simulink model "teach_from_joints"  (R2021a)
settings: Solver=FixedStepAuto  StartTime=0.0  StopTime=1000  FixedStep=SAMPLE_TIME  RelTol=1e-3
values from neighbouring files (symbols this model uses):
  dh_a = dh_list(:,3)    [move_joints_setup.m]
  dh_alpha = dh_list(:,4)    [move_joints_setup.m]
  dh_d = dh_list(:,2)+[0 0 0 0 0 length_f2t]'    [move_joints_setup.m]
  dh_theta_offset = dh_list(:,1)    [move_joints_setup.m]
  init_position = [274.5 0 543.1-138]    [move_joints_setup.m]
  initial_q = [0, 0, 0, 0, pi/2, 0]    [move_joints_setup.m]
  SAMPLE_TIME = 0.004    [move_joints_setup.m]
  theta_acc_max = theta_vel_max*2    [move_joints_setup.m]
  theta_max = [180,	80, 	70,     180,	110,	360]*pi/180    [move_joints_setup.m]
  theta_min = [-180,	-120,     -100,	-195,	-120,	-360]*pi/180    [move_joints_setup.m]
  theta_vel_max = [15, 10, 10, 40, 40, 40]*pi/180    [move_joints_setup.m]
undefined symbols (not defined in the file or in its folder): Px, Py, Pz, X, Y, Z
libraries: sm_lib x70, simulink x12, nesl_utility x11, dspswit3 x3, simulink_extras x2, sldrtlib x1, aerolibanimutils x1
(part 3 of 3)

== matlab function teach_from_joints/traj_planing/joint_traj/inver_kinematic2/inver_kinematic ==
  data: target input size=[4 4]; last_theta input size=[1 6]; a2 input; a3 input; flag output; possible_solv_num output; a4 input; final_theta output size=[1 6]; d1 input; d4 input; d6 input; theta_min input size=[1 6]; theta_max input size=[1 6]
function  [flag, possible_solv_num, final_theta]  = inver_kinematic_pack(target, last_theta, a2, a3, a4, d1, d4, d6, theta_min, theta_max)
%*****************************************************
%功能：给定目标位姿求出关节解
%这个求解函数必须满足dh参数中的关节角偏移量为：
%theta_offset = [0, -pi/2, 0, 0, 0, 0];
%和alpha = [0, -pi/2,  0, -pi/2, pi/2, -pi/2];这一条件，否则不适用。
%输入参数格式：1.target表示目标位姿，为4×4矩阵
%              2.robot_param 表示机器人参数，只针对特定机器人。格式为：
%                robot_param = [0 0; 0 a2; 0 a3; d4 a4; 0 0; d6 0];
%              3.joint_limit表示关节限制。格式为：joint_limit =[最小角度 最大角度 最大步长]
%               joint_limit = [theta1_min theta1_max theta1_step;……theta6_min theta6_max theta6_step];
%              4.last_theta表示机器人上一时刻各关节位置，该值用于筛选最优的关节角。格式为：
%               last_theta = [theta1, theta2, ……theta6]
%输出参数格式：1.flag:是否有解标志。1：表示有解；0表示无解。
%              2.final_theta表示最优的解，无解时为空矩阵final_theta = []
%               final_theta = [theta1, theta2, ……theta6]
%              3.all_theta 表示所有可能解,每一行表示一种可能解，最多有8种解。
%*****************************************************
    
%定义theta的第i行都是theta(i)的各种可能值
    joint_limit = [ theta_min', theta_max'];
    theta = zeros([6,8]);
    solvable_flag = bin2dec('00000000');    
%需要上一时刻机器关节角作为参考位形，用于筛选出最优解
    temp_last_theta = last_theta'; 
%当关节5为0时，设置关节4的值。
    theta4_variable = last_theta(4);
%建一个空矩阵，用于重新排列theta矩阵
%     t_1 = []; t_2 = []; t_3 = [];t_4 = []; t_5 = []; t_6 = []; 
    t_1 = zeros(1, 8);
    t_2 = zeros(1, 8);
    t_3 = zeros(1, 8);
    t_4 = zeros(1, 8);
    t_5 = zeros(1, 8);
    t_6 = zeros(1, 8);
    possible_solv_num = 0;
%换另一种表示法。
    %T_0_6 = [target.n, target.o, target.a,target.t];
    d1 = 0;
    target(3,4)=target(3,4)-0.3855-0.02;
    T_0_6 = target;
    d = [d1; 0; 0; d4; 0; d6];            %操作臂偏距
    a = [ 0;a2; a3; a4; 0; 0];            %操作臂偏距
    %腕关节的位姿。
    T_6_W = [1 0 0 0; 0 1 0 0; 0 0 1 -d(6); 0 0 0 1];
    T_0_W = T_0_6 * T_6_W;
    i1 = 1; i2 = 1; i3 = 1; i4 = 1; i5 = 1; i6 = 1; 
%因为theta1有两种可能
  for num_1 = 1:2
 %********************* theta1 *****************************
    temp_s1 = T_0_W(2,4);
    temp_c1 = T_0_W(1,4);
    temp_sgn = (-1)^num_1;
    theta(1, i1) = atan2(temp_sgn * temp_s1, temp_sgn * temp_c1);
    sin_1 = sin( theta(1, i1) );
    cos_1 = cos( theta(1, i1) );
 %********************* theta3 *****************************  
    temp_K1 = T_0_W(1,4)*cos_1 - a(2) + T_0_W(2,4)*sin_1;
    temp_K2 = T_0_W(3,4); 
    temp_K = (temp_K1^2 + temp_K2^2 - a(4)^2 - a(3)^2 - d(4)^2) / (2*a(3)); 
    temp_in_sqrt = a(4)^2 + d(4)^2 - temp_K^2;
    if  temp_in_sqrt >= 0
        %设置对应标志位位置1，表明这种情况可解。
        %如果solvable_flag ='00000001'说明第一种theta1有解；
        %如果solvable_flag='00000010'说明第二种theta1有解；
        %如果solvable_flag='00000011'说明两种theta1都有解；
        %如果solvable_flag ='00000000'说明目标点不在工作空间；
        solvable_flag = bitset(solvable_flag, num_1, 1);     
    end
%theta3有两种可能.
    for num_3 = 1:2  
        if  temp_in_sqrt < 0
            break;                                   %直接跳出 theta3无解
        else
            theta(3, i3) = atan2(a(4), d(4)) - atan2(temp_K, (-1)^(num_3)*sqrt(temp_in_sqrt));
        end
        sin_3 = sin(theta(3, i3));
        cos_3 = cos(theta(3, i3));
 %********************* theta2 *****************************  
        m1 = a(4)*cos_3-d(4)*sin_3+a(3);
        m2 = -a(4)*sin_3-d(4)*cos_3;
        temp_sin2 = m2*temp_K1-m1*temp_K2;
        temp_cos2 = temp_K1*m1+temp_K2*m2;
%         if temp_sin2 < 0
%             temp_sin2 = -temp_sin2;
%         end
%         if temp_cos2 < 0
%             temp_cos2 = -temp_cos2;
%         end
        theta(2, i2) = atan2(temp_sin2,temp_cos2);   
        sin_2 = sin(theta(2, i2));    %不能直接用temp_sin2，因为它不等于sin_2,少了一个分母。
        cos_2 = cos(theta(2, i2));
%********************* theta4 、theta5、theta6*****************************  
%求theta5
%             temp_3_3 =  aw(1)*(cos_1*cos_2*cos_3 - cos_1*sin_2*sin_3)...
%                         + aw(2)*(cos_2*cos_3*sin_1 - sin_1*sin_2*sin_3) ...
%                         - aw(3)*(cos_3*sin_2 + cos_2*sin_3);
            temp_2_3 = - T_0_W(3,3)*(cos_2*cos_3 - sin_2*sin_3) ...
            - T_0_W(1,3)*cos_1*(cos_2*sin_3 + cos_3*sin_2) ...
            - T_0_W(2,3)*sin_1*(cos_2*sin_3 + cos_3*sin_2);
%求theta4
%             temp_1_3 = aw(3)*(cos_2*cos_3 - sin_2*sin_3)...
%                         + aw(1)*(cos_1*cos_2*sin_3 + cos_1*cos_3*sin_2)...
%                         + aw(2)*(cos_2*sin_1*sin_3 + cos_3*sin_1*sin_2);
%             temp_3_3 =  aw(1)*sin_1 - aw(2)*cos_1;  
            temp_1_3 = T_0_W(1,3)*cos_1*(cos_2*cos_3 - sin_2*sin_3) ...
            - T_0_W(3,3)*(cos_2*sin_3 + cos_3*sin_2) ...
            + T_0_W(2,3)*sin_1*(cos_2*cos_3 - sin_2*sin_3);
            temp_3_3 = T_0_W(2,3)*cos_1 - T_0_W(1,3)*sin_1;
%求theta6
%             temp_3_1 =  nw(1)*(cos_1*cos_2*cos_3- cos_1*sin_2*sin_3)...
%                         + nw(2)*(cos_2*cos_3*sin_1 - sin_1*sin_2*sin_3)...
%                         - nw(3)*(cos_3*sin_2+cos_2*sin_3);            
%             temp_3_2 =  ow(1)*(cos_1*cos_2*cos_3- cos_1*sin_2*sin_3)...
%                         + ow(2)*(cos_2*cos_3*sin_1 - sin_1*sin_2*sin_3)...
%                         - ow(3)*(cos_3*sin_2+cos_2*sin_3); 
            temp_2_1 = - T_0_W(3,1)*(cos_2*cos_3 - sin_2*sin_3) ...
            - T_0_W(1,1)*cos_1*(cos_2*sin_3 + cos_3*sin_2) ...
            - T_0_W(2,1)*sin_1*(cos_2*sin_3 + cos_3*sin_2);
            temp_2_2 = - T_0_W(3,2)*(cos_2*cos_3 - sin_2*sin_3) ...
            - T_0_W(1,2)*cos_1*(cos_2*sin_3 + cos_3*sin_2) ...
            - T_0_W(2,2)*sin_1*(cos_2*sin_3 + cos_3*sin_2);
 %求theta4 + theta6                 
%             temp_1_1 = nw(3)*(cos_2*cos_3 - sin_2*sin_3)...
%                         + nw(1)*(cos_1*cos_2*sin_3 + cos_1*cos_3*sin_2)...
%                         + nw(2)*(cos_2*sin_1*sin_3+ cos_3*sin_1*sin_2);
%             temp_2_1 = nw(1)*sin_1 - nw(2)*cos_1; 
            temp_1_1 = T_0_W(1,1)*cos_1*(cos_2*cos_3 - sin_2*sin_3) ...
            - T_0_W(3,1)*(cos_2*sin_3 + cos_3*sin_2) ...
            + T_0_W(2,1)*sin_1*(cos_2*cos_3 - sin_2*sin_3);
            temp_1_2 = T_0_W(1,2)*cos_1*(cos_2*cos_3 - sin_2*sin_3) ...
            - T_0_W(3,2)*(cos_2*sin_3 + cos_3*sin_2) ...
            + T_0_W(2,2)*sin_1*(cos_2*cos_3 - sin_2*sin_3);
            
%判断theta5是否趋于零，如果它趋于零，则意味则temp_2_1 和temp_1_3都
%是趋于零的，因而theta4的方向可以任意取。并且轴4和轴6在一条直线上。
%根据theta5的正负号，cos(theta5)都是一样的，但是sin(theta5)却有正负之分。
%因此，theta4应该有两种情况，两者相差180度。
%1.theta5 < 0时， atan2(-temp_3_3, temp_1_3) 
%2.theta5 > 0时， atan2(temp_3_3, -temp_1_3)

%*****************     情况1      ****************
            threshold = 1.0e-14;
            for  num_5 = 1:2
                    temp_eq_1 = abs(temp_2_3 - 1);
                    if temp_eq_1 < threshold
                        theta(5, i5) = 0;
                    else
                        theta(5, i5) = acos(temp_2_3) * (-1)^(num_5);
                    end
                    %***********theta4 、theta6***************
                    if  -threshold < theta(5, i5) && theta(5, i5) < threshold   
                        temp_4and6 = atan2(-temp_1_2, temp_1_1);                 %这里暂时不考虑+2k*pi             
                        theta(4, i4) = theta4_variable;                         %这个可以任意取值。
                        theta(6, i6) = temp_4and6 - theta(4, i4); 
                        theta(6, i6) = correct_theta6(theta(6, i6), joint_limit(6, 1), joint_limit(6, 2)); %这里考虑+2k*pi
                    elseif theta(5, i5) <= -threshold
                        theta(4, i4) = atan2(-temp_3_3, temp_1_3);
                        theta(6, i6) = atan2(temp_2_2, -temp_2_1);
                    elseif theta(5, i5) >= threshold 
                        theta(4, i4) = atan2(temp_3_3, -temp_1_3);
                        theta(6, i6) = atan2(-temp_2_2, temp_2_1);
                    end
                    %真正存在的theta值。
                    possible_solv_num = possible_solv_num + 1;
                    t_1(possible_solv_num) = theta(1, i1);
                    t_2(possible_solv_num) = theta(2, i2);
                    t_3(possible_solv_num) = theta(3, i3);
                    t_4(possible_solv_num) = theta(4, i4);
                    t_5(possible_solv_num) = theta(5, i5);
                    t_6(possible_solv_num) = theta(6, i6);
                   %改变i4~i6，以便增加另外一个值。
                    i5 = i5 + 1;
                    i4 = i4 + 1;
                    i6 = i6 + 1;
            end
            i3 = i3 +1;
            i2 = i2 +1;
    end
    i1 = i1 + 1;
  end
%theta矩阵的格式不对，需要调整。
   theta_array = [t_1; t_2; t_3; t_4; t_5; t_6];
%筛选最优解出来。
    final_theta = zeros(1,6);
   if solvable_flag ~= 0
       [flag, final_theta] = choose_pretty(theta_array, possible_solv_num, joint_limit, temp_last_theta);   
%        if flag == 0
%            final_theta = last_theta;
%        end
   else
       final_theta = last_theta;
       flag = 0;
   end
   
end

function  output = correct_theta6(input, min, max)
    %给角度限制值加入一个计算精度误差computational accuracy =0.0001，
    temp_acc = 1e-4;
    if input < (min - temp_acc)
        output = input + 2*pi;
    elseif  input > (max + temp_acc)
        output = input - 2*pi;
    else
        output = input;
    end
end

function [flag, final_theta] = choose_pretty(theta, len, joint_limit, last_theta)
    %筛选1.结构限制2.位置变动最小第7行是距离和，第八行是最小行标志（不是最小行的置为0，是最小行的置为1）。
    distance = zeros(7, len);
   %最小的距离和 最小的角度，最小的大关节角度
    min_dis_sum = 1000;
    min_dis_num = 0;

    for possible_num = 1:len
        jump = 0;
        %********1.筛选符合关节限制范围内的,并计算关节角度变化的平方和。*************
        for joint_num = 1:6
            if theta(joint_num, possible_num) < (joint_limit(joint_num, 1) - 1e-4) || theta(joint_num, possible_num) > (joint_limit(joint_num, 2) + 1e-4)
                distance(7, possible_num) = 10000;
                jump = 1;
                break;
            else
                %角度变化量。
                temp_dis = abs(theta(joint_num, possible_num) -  last_theta(joint_num));
                distance(joint_num, possible_num) = temp_dis * temp_dis;    %求平方
                distance(7, possible_num) = distance(7, possible_num) + distance(joint_num, possible_num); %求和
            end
        end
        %*****************************结束筛选1*******************************
        
        %*************2.满足关节角度限制的,则筛选最小的总角度的。*********
        if jump == 0                 
            if min_dis_num == 0     %至少找的一个满足角度限制的，所以赋值给它。
                min_dis_num = possible_num;
            end

            if min_dis_sum < distance(7, possible_num)
                temp_min_sum = min_dis_sum;
            else
                temp_min_sum = distance(7, possible_num);
            end
            
            %找出最小的角度和对应编号。
            if (temp_min_sum ~= min_dis_sum)                        %如果不相等，意味着找到一个更小的。
                min_dis_sum = distance(7, possible_num);
                min_dis_num = possible_num;
            elseif distance(7, possible_num) == temp_min_sum        %如果最小值和新的值相等
                %**************3.再比较找出大关节运动最小******************
                for joint_num = 1:6
                    
                    if distance(joint_num, possible_num) < distance(joint_num, min_dis_num)
                        temp_min_joint = distance(joint_num, possible_num);
                    else
                        temp_min_joint = distance(joint_num, min_dis_num);
                    end

                    if temp_min_joint ~= distance(joint_num, min_dis_num) %找到一个动大关节更小的，直接跳出。
                        min_dis_num = possible_num;
                        break;
                    end
                end             
                %*********************结束筛选3********************************
            end
        end
       %****************************结束筛选2*****************************
    end
    
    if min_dis_num ~= 0     %
       temp_final_theta = theta(:, min_dis_num);
       flag = 1;
    else
       temp_final_theta = last_theta; 
       flag = 0;
    end
    final_theta = temp_final_theta';      %转置，写成行向量形式。
    final_theta(2) = final_theta(2) + pi/2;
end

== matlab function teach_from_joints/traj_planing/joint_traj/xyzrpy2matr ==
  data: position input size=[1 3]; T output size=[4 4]; angle input size=[1 3]
function T = xyzrpy2matr( position, angle)
    M = zeros(4, 4);
    R = angle(1);
    P = angle(2);
    Y = angle(3);
    C_R = cos(R); S_R = sin(R);
    C_P = cos(P); S_P = sin(P);
    C_Y = cos(Y); S_Y = sin(Y);
    %%
    %旋转矩阵
    rotate_x = [1       0       0
                0       C_R     -S_R
                0       S_R     C_R];  

    rotate_y = [C_P     0       S_P
                0       1       0
                -S_P    0       C_P];  
            
    rotate_z = [C_Y     -S_Y	0
                S_Y     C_Y     0
                0       0       1];          
    M(1:3, 1:3) = rotate_x * rotate_y * rotate_z;
    M(1:3, 4) = position';
    M(4, :) = [0, 0, 0, 1]; 
    T = M;
end

== matlab function teach_from_joints/traj_planing/joint_traj/joint_traj_sub/decelerate/limit_qd ==
  data: qd_input input size=[1, 6]; qd_output output size=[1, 6]; last_qd input size=[1, 6]; qd_max input size=[1, 6]; qdd_max input size=[1, 6]; dt input; percent_min output
function [qd_output, percent_min] = limit_qd( qd_input, last_qd, qd_max, qdd_max, dt)
%%使用伪逆矩阵求解，避免奇异点问题。
    threshold = abs(qdd_max * dt);
    threshold_N1 = 1;
    threshold_N2 = 10000;
    %%
    temp_qd = qd_input';
    temp_delta_qd = temp_qd - last_qd';
    temp_delta_qd_abs = abs(temp_delta_qd);
    temp_delta_qd_abs_limit = temp_delta_qd_abs;

    percent = ones(6,1);
    singula_flag = zeros(1,6);
    percent_min = 1;
%%
    for i = 1:6

        if temp_delta_qd_abs(i) > (threshold_N2*threshold(i))
            singula_flag(i) = 1;
            temp_delta_qd_abs(i) = threshold_N2*threshold(i);
        end
%限制速度值步长        
        if temp_delta_qd_abs(i) > (threshold_N1*threshold(i))
            temp_delta_qd_abs_limit(i) = threshold_N1*threshold(i);
            percent(i) = temp_delta_qd_abs_limit(i)/temp_delta_qd_abs(i);
        end
%加速步长百分比的最小值
        if percent(i) < percent_min
            percent_min = percent(i);
        end
    end
%%
%奇异点问题处理 
        delta_qd_out = sign(temp_delta_qd) .* temp_delta_qd_abs * percent_min;
        qd_output = delta_qd_out' + last_qd;
%%
    percent_qd = abs(qd_output./qd_max);
    percent_qd_max = max(percent_qd);
    if percent_qd_max > 1
        qd_output = qd_output / percent_qd_max;
    end
end

== matlab function teach_from_joints/traj_planing/joint_traj/joint_traj_sub/six_dof_traj_trape ==
  data: x0 input size=[1 6]; flag output; v0 input size=[1 6]; xf input size=[1 6]; vf input size=[1 6]; vMax input size=[1 6]; aMax input size=[1 6]; t input; xt output size=[1 6]; vt output size=[1 6]
function [flag, xt, vt] = traj_trape( x0,v0,xf,vf,vMax,aMax, t )
    %如果误差很小表示已经到达目标点。
    equal_1 = sum(abs(x0 - xf)) < 0.0001;
    equal_2 = sum(abs(v0 - zeros(1,6))) < 0.0001;
    equal_3 = sum(abs(vf - zeros(1,6))) < 0.0001;
    if equal_1 && equal_2 && equal_3
        flag = 1;
        xt = xf;
        vt = zeros(1,6);
        return;
        
    end
    [flag, xt, vt, test] = six_dof_traj( x0,v0,xf,vf,vMax,aMax, t );
end

function [flag, xt, vt,test ] = six_dof_traj( x0,v0,xf,vf,vMax,aMax, t )
%SIX_DOF_TRAJ 
%   此处显示详细说明
%
len =length(x0);

bangBangBool = zeros(1,len);
a0 = zeros(1,len);
b0 = zeros(1,len);
c0 = zeros(1,len);
a1 = zeros(1,len);
b1 = zeros(1,len);
a2 = zeros(1,len);
b2 = zeros(1,len);
c2 = zeros(1,len);
t1 = zeros(1,len);
t2 = zeros(1,len);
tf = zeros(1,len);
reach_flag = zeros(1,len);

v_use = vMax;
a_use = aMax;

t_max = 0;
plotBool = 0;
%%
%computer trajectory
for n = 1:2
    for i = 1:len
        [bangBangBool(i),a0(i),b0(i),c0(i),a1(i),b1(i),a2(i),b2(i),c2(i),t1(i),t2(i),tf(i)] = getMinTimeTrajCoeffs(x0(i),v0(i),xf(i),vf(i),v_use(i),a_use(i));
        if tf(i) > t_max
            t_max = tf(i);
        end
    end
    %第二次就直接跳出了
    if n==2
        break;
    end
    
    v_use = abs(xf - x0)/t_max;
    for i = 1:len
        if v_use(i) < abs(v0(i))
            v_use(i) = abs(v0(i));
        end
    end
    a_use = (aMax./vMax) .* v_use;
end
%%
%ouput_value
xt = ones(1,len);
vt = ones(1,len);

for i = 1:len
    if bangBangBool(i) == 0     %have line
        if t<t1(i)
         	xt(i) = a0(i) + b0(i)*t + c0(i)*t^2;
            vt(i) = b0(i) + 2*c0(i)*t;
        elseif  t <=t2(i)
            xt(i) = a1(i) + b1(i)*t;
            vt(i) = b1(i);
        elseif t <= tf(i)
            xt(i) = a2(i) + b2(i)*t + c2(i)*t^2;
            vt(i) = b2(i) + 2*c2(i)*t;
        else
            xt(i) = xf(i);
            vt(i) = vf(i);
            reach_flag(i) = 1;
        end
        test = 100;
    else                        %have not line
        if t<=t2(i)
         	xt(i) = a0(i) + b0(i)*t + c0(i)*t^2;
            vt(i) = b0(i) + 2*c0(i)*t;
        elseif t <= tf(i)
            xt(i) = a2(i) + b2(i)*t + c2(i)*t^2;
            vt(i) = b2(i) + 2*c2(i)*t;
        else
            xt(i) = xf(i);
            vt(i) = vf(i);
            reach_flag(i) = 1;
        end
        test = 200;
    end 
%  test = tf(1);  

end

%%
% judge whether reach target
for i = 1:len
    if reach_flag(i) ~= 1
        flag = 0;
        break;
    end
    flag = 1;
end
end

%
% single dof traj
% 
function [bangBangBool,a0,b0,c0,a1,b1,a2,b2,c2,t1,t2,tf] = getMinTimeTrajCoeffs(x0,v0,xf,vf,vMax,aMax)
% Calculate the coefficients that define the three segments of an LSPB
% trajectory between state [x0,v0] and [xf,vf]. This code assumes maximum speed and
% acceleration are independent of direction.  Note that the acceleration is
% either -aMax, 0, or aMax at all times.  The resulting LSPB trajectory is
% the fastest trajectory possible that meets these velocity and
% acceleration constraints.

% Input:
%       x0: Initial position
%       v0: Initial velocity
%       xf: Final position
%       vf: Final velocity
%       vMax: Maximum allowed speed (either direction)
%       aMax: Maximum allowed acceleration (either direction)
%       plotBool: Set to 1 to generate a simple plot of the LSPB

% Output:
%       bangBangBool: 0 indicates that the trajectory contains a linear
%           portion, meaning all coefficients and output t's are required.
%           1 indicates that a linear portion is not required, thus the a1,
%           b1, and t1 output values will all be zero and can be ignored.
%       a0,b0,c0: Define first segment of LSPB (parabolic).  
%           For 0<=t<=t1, x = a0 + b0*t + c0*t^2
%       a1,b1: Define second segment of LSPB (linear).  
%           For t1<=t<=t2, x = a1 + b1*t 
%       a2,b2,c2: Define third segment of LSPB (parabolic).  
%           For t2<=t<=tf, x = a2 + b2*t + c2*t^2
%       t1,t2,tf: Times at which the above equations hold.

% Eric Young, 2018

%Check for errors
if(0>vMax)
    error('vMax must be positive')
end
if(0>aMax)
    error('aMax must be positive')
end
if(v0>vMax)
    error('Initial velocity is greater than vMax')
end
if(v0<-vMax)
    error('Initial velocity is less than -vMax')
end
if(vf>vMax)
    error('Final velocity is greater than vMax')
end
if(vf<-vMax)
    error('Final velocity is less than -vMax')
end


% First calculate maximum distance possible without linear segment
xfMaxBangBang = x0 + (vMax^2 - v0^2)/(2*aMax) + (vMax^2 - vf^2)/(2*aMax);

% Distance with only one parabolic blend (later used to determine if the
% first parabolic segment should have positive or negative
% acceleration)
if(vf>=v0)
    xfBang = x0 + (vf^2 - v0^2)/(2*aMax);
else
    xfBang = x0 + (v0^2 - vf^2)/(2*aMax);%xfBang = x0 + (vf^2 - v0^2)/(2*-aMax);
end

% Minimum distance possible without linear segment
xfMinBangBang = x0 + (vMax^2 - v0^2)/(2*-aMax) + (vMax^2 - vf^2)/(2*-aMax);

% Determine acceleration for first segment.  n = 1: begin with positive
% acceleration
if(xf>xfMaxBangBang)
    n = 1;
    bangBangBool = 0;
elseif(xf<xfMinBangBang)
    n = -1;
    bangBangBool = 0;
else
    bangBangBool = 1;
    if(xf>=xfBang)
        n = 1;
    else
        n = -1;
    end
end

% True for all cases
a0 = x0;
b0 = v0;
c0 = n*aMax/2;
c2 = -n*aMax/2;

%If no linear segment is needed (just a bang-bang trajectory)
if(bangBangBool)
    % Ignore linear portion
    t1 = 0;
    a1 = 0;
    b1 = 0;
    
    m = sqrt(2*c0*(xf-x0)+v0^2/2+vf^2/2);
    t2 = (-b0+m)/(2*c0);
    b2 = b0+4*c0*t2;
    tf = (b0+4*c0*t2 - vf)/(2*c0);
    a2 = a0 + b0*t2 + c0*t2^2 - b2*t2 - c2*t2^2;  
    if(t2>tf)||(t2<0)
        t2 = (-b0 - m)/(2*c0);
        b2 = b0+4*c0*t2;
        tf = (b0+4*c0*t2 - vf)/(2*c0);
        a2 = a0 + b0*t2 + c0*t2^2 - b2*t2 - c2*t2^2; 
    end

else %LSPB bool = 1, linear segment is needed
    b1 = n*vMax;
    t1 = (n*vMax - b0)/(2*c0);
    a1 = a0 + b0*t1 + c0*t1^2 - b1*t1;
    t2 = (xf - a1 + (n^2*vMax^2)/(4*c2) - (vf^2)/(4*c2))/b1;
    tf = (2*c2*t2 + vf - n*vMax)/(2*c2);
    b2 = n*vMax - 2*c2*t2;
    a2 = xf - b2*tf - c2*tf^2;
    
end

end
